simulink library "INT_AccPed_DrvDemDes"  (R2016b)
settings: Solver=VariableStepAuto  StartTime=0.0  StopTime=10.0  RelTol=1e-3
settings Model: Creator=bianxuyin  LastModifiedBy=bianxuyin

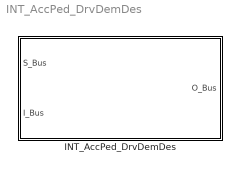
== system INT_AccPed_DrvDemDes ==
  INT_AccPed_DrvDemDes : Subsystem

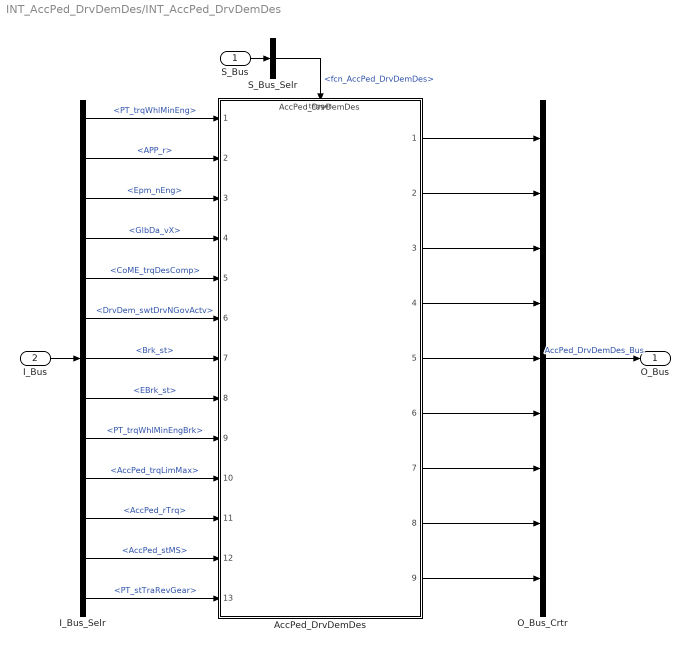
== system INT_AccPed_DrvDemDes/INT_AccPed_DrvDemDes ==
  S_Bus : Inport
  I_Bus : Inport  Port=2
  AccPed_DrvDemDes : ModelReference  ModelNameDialog=AccPed_DrvDemDes  SimulationMode=Normal  ModelReferenceVersion=1.65  TriggerPortName=function  TriggerPortTriggerType=function-call  TriggerPortStatesWhenEnabling=held
  I_Bus_Selr : BusSelector  OutputSignals=PT_trqWhlMinEng,APP_r,Epm_nEng,GlbDa_vX,CoME_trqDesComp,DrvDem_swtDrvNGovActv,Brk_st,EBrk_st,PT_trqWhlMinEngBrk,AccPed_trqLimMax,AccPed_rTrq,AccPed_stMS,PT_stTraRevGear
  O_Bus_Crtr : BusCreator  Inputs=9
  S_Bus_Selr : BusSelector  OutputSignals=fcn_AccPed_DrvDemDes
  O_Bus : Outport
  wires:
  S_Bus_Selr/1 -> AccPed_DrvDemDes/Trigger  "<fcn_AccPed_DrvDemDes>"
  S_Bus/1 -> S_Bus_Selr/1
  I_Bus/1 -> I_Bus_Selr/1
  I_Bus_Selr/1 -> AccPed_DrvDemDes/1  "<PT_trqWhlMinEng>"
  I_Bus_Selr/2 -> AccPed_DrvDemDes/2  "<APP_r>"
  I_Bus_Selr/3 -> AccPed_DrvDemDes/3  "<Epm_nEng>"
  I_Bus_Selr/4 -> AccPed_DrvDemDes/4  "<GlbDa_vX>"
  I_Bus_Selr/5 -> AccPed_DrvDemDes/5  "<CoME_trqDesComp>"
  I_Bus_Selr/6 -> AccPed_DrvDemDes/6  "<DrvDem_swtDrvNGovActv>"
  I_Bus_Selr/7 -> AccPed_DrvDemDes/7  "<Brk_st>"
  I_Bus_Selr/8 -> AccPed_DrvDemDes/8  "<EBrk_st>"
  I_Bus_Selr/9 -> AccPed_DrvDemDes/9  "<PT_trqWhlMinEngBrk>"
  I_Bus_Selr/10 -> AccPed_DrvDemDes/10  "<AccPed_trqLimMax>"
  I_Bus_Selr/11 -> AccPed_DrvDemDes/11  "<AccPed_rTrq>"
  I_Bus_Selr/12 -> AccPed_DrvDemDes/12  "<AccPed_stMS>"
  I_Bus_Selr/13 -> AccPed_DrvDemDes/13  "<PT_stTraRevGear>"
  O_Bus_Crtr/1 -> O_Bus/1  "AccPed_DrvDemDes_Bus"
  AccPed_DrvDemDes/1 -> O_Bus_Crtr/1
  AccPed_DrvDemDes/2 -> O_Bus_Crtr/2
  AccPed_DrvDemDes/3 -> O_Bus_Crtr/3
  AccPed_DrvDemDes/4 -> O_Bus_Crtr/4
  AccPed_DrvDemDes/5 -> O_Bus_Crtr/5
  AccPed_DrvDemDes/6 -> O_Bus_Crtr/6
  AccPed_DrvDemDes/7 -> O_Bus_Crtr/7
  AccPed_DrvDemDes/8 -> O_Bus_Crtr/8
  AccPed_DrvDemDes/9 -> O_Bus_Crtr/9
